simulink model "simula_PI_D_discreto"  (R2017a)
settings: Solver=FixedStepAuto  StartTime=0.0  StopTime=4000  FixedStep=Tc  RelTol=1e-3
values from neighbouring files (symbols this model uses):
  a1 = .5    (= 0.5)    [metodo_grafico.m]
  a2 = .5    (= 0.5)    [metodo_grafico.m]
  b1 = (Td - 2*N*Tc)/(Td + 2*N*Tc)    [metodo_grafico.m]
  b2 = -(2*kP*Td*N)/(Td+2*N*Tc)    [metodo_grafico.m]
  Tc = 1.5    [metodo_grafico.m]
undefined symbols (not defined in the file or in its folder): kP, Ti
libraries: cstblocks x1
settings Model: Creator=Enrico Donato  LastModifiedBy=Enrico Donato

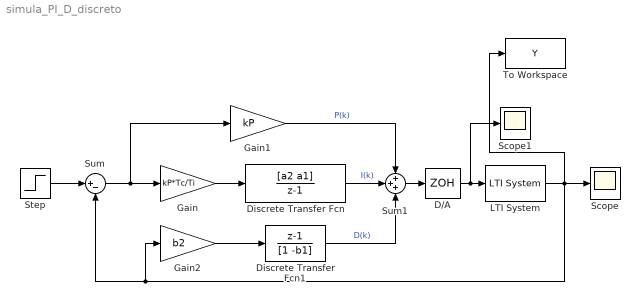
== system simula_PI_D_discreto ==
  D/A : ZeroOrderHold  SampleTime=-1
  Discrete Transfer Fcn : DiscreteTransferFcn  Numerator=[a2 a1]  Denominator=[1 -1]  SampleTime=Tc
  Discrete Transfer Fcn1 : DiscreteTransferFcn  Numerator=[1 -1]  Denominator=[1 -b1]  SampleTime=Tc
  Gain : Gain  Gain=kP*Tc/Ti
  Gain1 : Gain  Gain=kP
  Gain2 : Gain  Gain=b2
  LTI System : cstblocks/LTI System  sys=G  IC=[]
  Scope : Scope
  Scope1 : Scope
  Step : Step  SampleTime=0
  Sum : Sum  Inputs=|+-
  Sum1 : Sum  Inputs=+++
  To Workspace : ToWorkspace  VariableName=Y  SampleTime=-1
  wires:
  Sum/1 -> Gain1/1, Gain/1
  Gain/1 -> Discrete Transfer Fcn/1
  Discrete Transfer Fcn/1 -> Sum1/2  "I(k)"
  Gain1/1 -> Sum1/1  "P(k)"
  LTI System/1 -> To Workspace/1, Scope/1, Sum/2, Gain2/1
  Gain2/1 -> Discrete Transfer Fcn1/1
  Discrete Transfer Fcn1/1 -> Sum1/3  "D(k)"
  Step/1 -> Sum/1
  Sum1/1 -> D/A/1
  D/A/1 -> Scope1/1, LTI System/1
